simulink model "GPCA_AlarmNoActions"  (Simulink 9.0)
settings: Solver=FixedStepDiscrete  StartTime=0.0  StopTime=19.8  FixedStep=0.200000  RelTol=1e-3  EnableMultiTasking=on
model workspace (MAT data in the model file):
  already_pp = 1
  input_struct.time = [0; 0.2; 0.4; 0.6; 0.8; 1; 1.2; 1.4; 1.6; 1.8; 2; 2.2; 2.4; 2.6; 2.8; 3; 3.2; 3.4; 3.6; 3.8; 4; 4.2; 4.4; 4.6; 4.8; 5; 5.2; 5.4; 5.6; 5.8; 6; 6.2; 6.4; 6.6; 6.8; 7; 7.2; 7.4; 7.6; 7.8; 8; 8.2; 8.4; 8.6; 8.8; 9; 9.2; 9.4; 9.6; 9.8; 10; 10.2; 10.4; 10.6; 10.8; 11; 11.2; 11.4; 11.6; 11.8; 12; 12.2; 12.4; 12.6; 12.8; 13; 13.2; 13.4; 13.6; 13.8; 14; 14.2; 14.4; 14.6; 14.8; 15; 15.2; 15.4; 15.6; 15.8; 16; 16.2; 16.4; 16.6; 16.8; 17; 17.2; 17.4; 17.6; 17.8; 18; 18.2; 18.4; 18.6; 18.8; 19; 19.2; 19.4; 19.6; 19.8]
  input_struct.signals(1).name = 'In1'
  input_struct.signals(1).values = [1; 0; 1; 0; 0; 1; 0; 1; 0; 1; 1; 1; 0; 1; 1; 0; 0; 1; 1; 0; 0; 0; 0; 0; 0; 0; 0; 0; 1; 0; 1; 0; 0; 0; 1; 1; 1; 1; 1; 0; 0; 0; 0; 1; 1; 1; 1; 0; 1; 1; 0; 1; 1; 1; 1; 0; 0; 1; 0; 1; 1; 1; 0; 0; 0; 0; 1; 1; 1; 0; 0; 1; 0; 1; 1; 0; 1; 1; 1; 1; 1; 1; 1; 1; 0; 0; 1; 1; 0; 1; 1; 1; 0; 1; 1; 1; 1; 0; 1; 0]
  input_struct.signals(1).dimensions = 1
  input_struct.signals(2).name = 'In2'
  input_struct.signals(2).values = [0; 1; 1; 1; 0; 1; 0; 1; 1; 1; 0; 0; 0; 1; 1; 1; 1; 1; 0; 1; 0; 0; 1; 1; 1; 0; 1; 1; 0; 0; 0; 1; 0; 1; 1; 0; 0; 1; 1; 1; 1; 0; 0; 1; 1; 1; 0; 1; 0; 0; 0; 1; 0; 0; 0; 0; 1; 1; 0; 0; 1; 1; 1; 1; 0; 1; 0; 0; 0; 0; 0; 0; 0; 1; 0; 0; 1; 1; 1; 1; 1; 1; 1; 0; 0; 0; 0; 1; 0; 0; 1; 0; 1; 1; 1; 1; 0; 0; 1; 1]
  input_struct.signals(2).dimensions = 1
  input_struct.signals(3).name = 'In3'
  input_struct.signals(3).values = [1; 1; 1; 1; 0; 0; 0; 1; 1; 1; 1; 0; 1; 1; 0; 1; 1; 0; 1; 1; 0; 0; 0; 1; 1; 0; 1; 1; 1; 1; 0; 0; 1; 0; 0; 0; 1; 0; 1; 0; 1; 0; 0; 1; 0; 1; 1; 0; 0; 0; 0; 0; 1; 1; 1; 1; 0; 1; 0; 1; 0; 1; 0; 1; 1; 1; 1; 1; 0; 0; 1; 1; 1; 0; 1; 1; 0; 1; 1; 0; 1; 1; 0; 1; 1; 1; 1; 0; 0; 1; 1; 0; 0; 0; 0; 0; 1; 0; 0; 0]
  input_struct.signals(3).dimensions = 1
  input_struct.signals(4).name = 'In4'
  input_struct.signals(4).values = [0; 0; 0; 0; 0; 0; 0; 0; 0; 1; 0; 1; 0; 0; 0; 0; 0; 0; 0; 0; 0; 0; 1; 1; 1; 0; 0; 0; 1; 0; 0; 0; 0; 0; 1; 0; 1; 1; 0; 1; 1; 1; 1; 0; 1; 0; 0; 1; 1; 0; 0; 1; 1; 1; 1; 0; 1; 0; 1; 0; 1; 1; 0; 0; 0; 0; 0; 1; 0; 1; 0; 0; 0; 0; 1; 1; 1; 1; 0; 0; 0; 0; 0; 1; 1; 1; 0; 0; 1; 1; 1; 1; 1; 1; 0; 1; 0; 0; 0; 0]
  input_struct.signals(4).dimensions = 1
  input_struct.signals(5).name = 'In5'
  input_struct.signals(5).values = [1; 0; 1; 0; 0; 1; 0; 1; 1; 0; 0; 1; 1; 1; 0; 0; 1; 1; 1; 1; 1; 0; 1; 0; 0; 1; 0; 1; 1; 0; 0; 0; 1; 0; 0; 0; 0; 0; 0; 0; 0; 1; 0; 1; 1; 0; 0; 1; 0; 0; 1; 0; 1; 1; 1; 1; 0; 1; 0; 1; 1; 1; 0; 0; 0; 1; 1; 1; 1; 0; 1; 1; 0; 1; 0; 0; 1; 0; 1; 1; 1; 1; 1; 1; 0; 0; 1; 0; 0; 0; 1; 1; 1; 0; 0; 1; 1; 1; 0; 0]
  input_struct.signals(5).dimensions = 1
  input_struct.signals(6).name = 'In6'
  input_struct.signals(6).values = [1; 1; 1; 0; 1; 0; 1; 0; 0; 0; 1; 1; 0; 0; 0; 1; 1; 0; 0; 0; 1; 1; 0; 0; 1; 0; 0; 1; 0; 1; 1; 1; 0; 1; 1; 0; 1; 0; 0; 0; 1; 1; 0; 1; 0; 1; 1; 0; 1; 0; 1; 0; 0; 1; 1; 0; 0; 1; 0; 1; 1; 1; 0; 0; 1; 1; 1; 1; 1; 0; 1; 0; 0; 0; 1; 1; 1; 1; 1; 1; 1; 0; 0; 0; 1; 1; 1; 1; 0; 1; 1; 0; 1; 0; 0; 0; 0; 1; 0; 0]
  input_struct.signals(6).dimensions = 1
  input_struct.signals(7).name = 'In7'
  input_struct.signals(7).values = [0; 0; 0; 1; 0; 0; 0; 1; 0; 1; 1; 0; 1; 1; 0; 1; 1; 0; 0; 1; 1; 1; 0; 1; 1; 1; 1; 0; 0; 0; 0; 0; 0; 1; 1; 0; 0; 0; 0; 0; 0; 1; 0; 1; 0; 0; 0; 0; 0; 1; 0; 1; 1; 1; 0; 0; 0; 1; 1; 0; 0; 1; 1; 0; 1; 1; 0; 1; 0; 0; 1; 1; 0; 1; 1; 1; 0; 0; 0; 1; 0; 0; 1; 1; 0; 0; 0; 1; 0; 0; 1; 0; 1; 1; 0; 0; 1; 1; 1; 1]
  input_struct.signals(7).dimensions = 1
  input_struct.signals(8).name = 'In8'
  input_struct.signals(8).values = [0; 1; 0; 0; 0; 1; 1; 1; 1; 0; 1; 0; 1; 1; 1; 0; 0; 1; 1; 1; 1; 1; 1; 1; 0; 1; 0; 0; 1; 0; 0; 1; 0; 0; 0; 0; 0; 1; 0; 0; 0; 0; 1; 0; 1; 1; 1; 1; 0; 0; 1; 0; 1; 1; 1; 0; 1; 0; 0; 0; 1; 1; 1; 1; 0; 1; 0; 1; 1; 1; 1; 1; 0; 0; 1; 0; 0; 0; 0; 1; 1; 1; 0; 1; 1; 1; 1; 0; 1; 0; 1; 1; 1; 0; 1; 0; 0; 1; 1; 0]
  input_struct.signals(8).dimensions = 1
  input_struct.signals(9).name = 'In9'
  input_struct.signals(9).values = [1; 1; 0; 0; 0; 0; 0; 1; 0; 1; 0; 1; 0; 1; 1; 0; 0; 0; 0; 0; 0; 1; 1; 1; 0; 1; 0; 1; 1; 0; 1; 1; 1; 1; 1; 0; 0; 0; 1; 1; 0; 0; 1; 1; 1; 0; 1; 1; 0; 0; 0; 1; 1; 0; 1; 1; 0; 0; 1; 1; 1; 1; 0; 0; 1; 1; 1; 0; 1; 1; 1; 0; 0; 1; 0; 1; 1; 0; 1; 0; 1; 0; 0; 1; 0; 0; 0; 0; 1; 1; 0; 0; 1; 0; 1; 1; 1; 1; 0; 1]
  input_struct.signals(9).dimensions : numeric (value not decoded)
settings Model: SuppressorTable=22 serialization::archive 11 0 6 0 0 0 0 0  Creator=bourbouh  LastModifiedBy=hbourbou
settings DataIOCC: ExternalInput=input_struct  LoadExternalInput=on  SaveFormat=Structure  SaveState=on
settings DebuggingCC: AlgebraicLoopMsg=error  ArtificialAlgebraicLoopMsg=error  UnderspecifiedInitializationDetection=Simplified  MergeDetectMultiDrivingBlocksExec=error  SingleTaskRateTransMsg=error
settings HardwareCC: ProdBitPerPointer=64  ProdBitPerSizeT=64  ProdBitPerPtrDiffT=64  ProdLargestAtomicFloat=Float  ProdIntDivRoundTo=Zero  ProdEndianess=LittleEndian  ProdWordSize=64  ProdHWDeviceType=Intel->x86-64 (Windows64)
settings ModelReferenceCC: PropagateSignalLabelsOutOfModel=on
settings GRTTargetCC: GeneratePreprocessorConditionals=Disable all  ExtMode=on

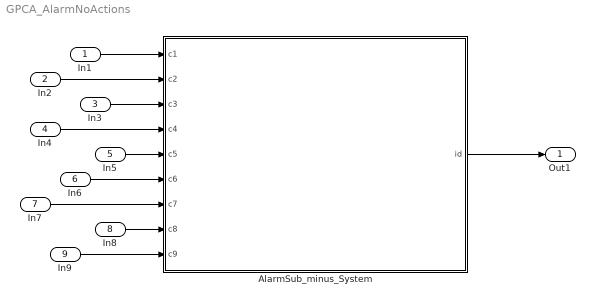
== system GPCA_AlarmNoActions ==
  In1 : Inport  OutDataTypeStr=boolean  PortDimensions=1
  In2 : Inport  Port=2  OutDataTypeStr=boolean  PortDimensions=1
  In3 : Inport  Port=3  OutDataTypeStr=boolean  PortDimensions=1
  In4 : Inport  Port=4  OutDataTypeStr=boolean  PortDimensions=1
  In5 : Inport  Port=5  OutDataTypeStr=boolean  PortDimensions=1
  In6 : Inport  Port=6  OutDataTypeStr=boolean  PortDimensions=1
  In7 : Inport  Port=7  OutDataTypeStr=boolean  PortDimensions=1
  In8 : Inport  Port=8  OutDataTypeStr=boolean  PortDimensions=1
  In9 : Inport  Port=9  OutDataTypeStr=boolean  PortDimensions=1
  AlarmSub_minus_System : Stateflow chart  TreatAsAtomicUnit=on
  Out1 : Outport
  wires:
  AlarmSub_minus_System/1(id) -> Out1/1
  In9/1 -> AlarmSub_minus_System/9(c9)
  In8/1 -> AlarmSub_minus_System/8(c8)
  In7/1 -> AlarmSub_minus_System/7(c7)
  In6/1 -> AlarmSub_minus_System/6(c6)
  In5/1 -> AlarmSub_minus_System/5(c5)
  In4/1 -> AlarmSub_minus_System/4(c4)
  In3/1 -> AlarmSub_minus_System/3(c3)
  In2/1 -> AlarmSub_minus_System/2(c2)
  In1/1 -> AlarmSub_minus_System/1(c1)

== stateflow chart AlarmSub_minus_System ==
  state Alarms
    state CheckAlarm [parallel]
      settings: executionOrder=1
      state CancelAlarm [parallel]
        settings: executionOrder=1
        state ON
          en: id = 2112;
        state OFF
          en: id = 2111;
        (default) -> Alarms.CheckAlarm.CancelAlarm.OFF
        Alarms.CheckAlarm.CancelAlarm.OFF -> Alarms.CheckAlarm.CancelAlarm.ON : [c5]
        Alarms.CheckAlarm.CancelAlarm.ON -> Alarms.CheckAlarm.CancelAlarm.OFF : [c4]
      state Level4 [parallel]
        settings: executionOrder=2
        state IsEmptyReservoir [parallel]
          settings: executionOrder=1
          state No
            en: id=21111;
          state Yes
            en: id=21112;
          (default) -> Alarms.CheckAlarm.Level4.IsEmptyReservoir.No [order 2]
          (default) -> Alarms.CheckAlarm.Level4.IsEmptyReservoir.Yes [order 1] : [c6]
          Alarms.CheckAlarm.Level4.IsEmptyReservoir.No -> Alarms.CheckAlarm.Level4.IsEmptyReservoir.Yes : [c7]
          Alarms.CheckAlarm.Level4.IsEmptyReservoir.Yes -> Alarms.CheckAlarm.Level4.IsEmptyReservoir.No [order 2] : [c8]
          Alarms.CheckAlarm.Level4.IsEmptyReservoir.Yes -> Alarms.CheckAlarm.Level4.IsEmptyReservoir.Yes [order 1] : [c9]
        state IsHardwareError [parallel]
          settings: executionOrder=2
          state Yes
            en: id=21122;
          state No
            en: id=21121;
          (default) -> Alarms.CheckAlarm.Level4.IsHardwareError.No [order 2]
          (default) -> Alarms.CheckAlarm.Level4.IsHardwareError.Yes [order 1] : [c3]
          Alarms.CheckAlarm.Level4.IsHardwareError.No -> Alarms.CheckAlarm.Level4.IsHardwareError.Yes : [c2]
          Alarms.CheckAlarm.Level4.IsHardwareError.Yes -> Alarms.CheckAlarm.Level4.IsHardwareError.No : [c4]
        state IsEnviromentalError [parallel]
          settings: executionOrder=3
          state Yes
            en: id=21132;
          state No
            en: id=21131;
          (default) -> Alarms.CheckAlarm.Level4.IsEnviromentalError.Yes [order 1] : [c6]
          (default) -> Alarms.CheckAlarm.Level4.IsEnviromentalError.No [order 2]
          Alarms.CheckAlarm.Level4.IsEnviromentalError.No -> Alarms.CheckAlarm.Level4.IsEnviromentalError.Yes : [c5]
          Alarms.CheckAlarm.Level4.IsEnviromentalError.Yes -> Alarms.CheckAlarm.Level4.IsEnviromentalError.No : [c7]
      state Level3 [parallel]
        settings: executionOrder=3
        state IsOverInfusionFlowRate [parallel]
          entry:id=21131;
          settings: executionOrder=1
          state Yes
            entry:id=21133;
          state Check
            entry:id=21132;
          state Monitor
            entry:id=21134;
          (default) -> Alarms.CheckAlarm.Level3.IsOverInfusionFlowRate.Check [order 3]
          (default) -> Alarms.CheckAlarm.Level3.IsOverInfusionFlowRate.Yes [order 1] : [c4]
          Alarms.CheckAlarm.Level3.IsOverInfusionFlowRate.Yes -> Alarms.CheckAlarm.Level3.IsOverInfusionFlowRate.Yes [order 1] : [c5]
          Alarms.CheckAlarm.Level3.IsOverInfusionFlowRate.Check -> Alarms.CheckAlarm.Level3.IsOverInfusionFlowRate.Yes [order 1] : [c6]
          Alarms.CheckAlarm.Level3.IsOverInfusionFlowRate.Yes -> Alarms.CheckAlarm.Level3.IsOverInfusionFlowRate.Check [order 2] : [c7]
          Alarms.CheckAlarm.Level3.IsOverInfusionFlowRate.Monitor -> Alarms.CheckAlarm.Level3.IsOverInfusionFlowRate.Yes [order 1] : [c7]
          Alarms.CheckAlarm.Level3.IsOverInfusionFlowRate.Monitor -> Alarms.CheckAlarm.Level3.IsOverInfusionFlowRate.Check [order 2] : [c9]
          Alarms.CheckAlarm.Level3.IsOverInfusionFlowRate.Check -> Alarms.CheckAlarm.Level3.IsOverInfusionFlowRate.Monitor [order 2] : [c8]
          Alarms.CheckAlarm.Level3.IsOverInfusionFlowRate.Monitor -> Alarms.CheckAlarm.Level3.IsOverInfusionFlowRate.Monitor [order 3] : [c8]
          (default) -> Alarms.CheckAlarm.Level3.IsOverInfusionFlowRate.Monitor [order 2] : [c4]
        state IsOverInfusionVTBI [parallel]
          settings: executionOrder=2
          state Yes
            en: id=211342
          state No
            en: id = 211341;
          (default) -> Alarms.CheckAlarm.Level3.IsOverInfusionVTBI.No [order 2]
          (default) -> Alarms.CheckAlarm.Level3.IsOverInfusionVTBI.Yes [order 1] : [c5]
          Alarms.CheckAlarm.Level3.IsOverInfusionVTBI.Yes -> Alarms.CheckAlarm.Level3.IsOverInfusionVTBI.Yes [order 1] : [c6]
          Alarms.CheckAlarm.Level3.IsOverInfusionVTBI.No -> Alarms.CheckAlarm.Level3.IsOverInfusionVTBI.Yes : [c7]
          Alarms.CheckAlarm.Level3.IsOverInfusionVTBI.Yes -> Alarms.CheckAlarm.Level3.IsOverInfusionVTBI.No [order 2] : [c8]
        state IsAirInLine [parallel]
          settings: executionOrder=3
          state Yes
            en: id=211332
          state No
            en: id = 211331;
          (default) -> Alarms.CheckAlarm.Level3.IsAirInLine.Yes [order 1] : [c1]
          (default) -> Alarms.CheckAlarm.Level3.IsAirInLine.No [order 2]
          Alarms.CheckAlarm.Level3.IsAirInLine.No -> Alarms.CheckAlarm.Level3.IsAirInLine.Yes : [c2]
          Alarms.CheckAlarm.Level3.IsAirInLine.Yes -> Alarms.CheckAlarm.Level3.IsAirInLine.No : [c3]
        state IsOcclusion [parallel]
          settings: executionOrder=4
          state Yes
            en: id=31132
          state No
            en: id=31131
          (default) -> Alarms.CheckAlarm.Level3.IsOcclusion.No [order 2]
          (default) -> Alarms.CheckAlarm.Level3.IsOcclusion.Yes [order 1] : [c7]
          Alarms.CheckAlarm.Level3.IsOcclusion.No -> Alarms.CheckAlarm.Level3.IsOcclusion.Yes : [c8]
          Alarms.CheckAlarm.Level3.IsOcclusion.Yes -> Alarms.CheckAlarm.Level3.IsOcclusion.No : [c9]
        state IsDoor_Open [parallel]
          settings: executionOrder=5
          state No
            en: id=32221
          state Yes
            en: id=32222
          (default) -> Alarms.CheckAlarm.Level3.IsDoor_Open.Yes [order 1] : [c1]
          (default) -> Alarms.CheckAlarm.Level3.IsDoor_Open.No [order 2]
          Alarms.CheckAlarm.Level3.IsDoor_Open.No -> Alarms.CheckAlarm.Level3.IsDoor_Open.Yes : [c2]
          Alarms.CheckAlarm.Level3.IsDoor_Open.Yes -> Alarms.CheckAlarm.Level3.IsDoor_Open.No : [c3]
      state Level2 [parallel]
        settings: executionOrder=4
        state IsLowReservoir [parallel]
          settings: executionOrder=1
          state No
            en: id = 42421;
          state Yes
            en: id=42422;
          (default) -> Alarms.CheckAlarm.Level2.IsLowReservoir.Yes [order 1] : [c5]
          (default) -> Alarms.CheckAlarm.Level2.IsLowReservoir.No [order 2]
          Alarms.CheckAlarm.Level2.IsLowReservoir.No -> Alarms.CheckAlarm.Level2.IsLowReservoir.Yes : [c6]
          Alarms.CheckAlarm.Level2.IsLowReservoir.Yes -> Alarms.CheckAlarm.Level2.IsLowReservoir.No : [c7]
      state Level1 [parallel]
        settings: executionOrder=5
        state IsUnderInfusion [parallel]
          entry: id=55111;
          settings: executionOrder=1
          state Yes
            entry:id=55113;
          state Check
            entry: id=55112;
          state Monitor
            entry: id=55114;
          (default) -> Alarms.CheckAlarm.Level1.IsUnderInfusion.Check [order 3]
          (default) -> Alarms.CheckAlarm.Level1.IsUnderInfusion.Yes [order 1] : [c1]
          Alarms.CheckAlarm.Level1.IsUnderInfusion.Check -> Alarms.CheckAlarm.Level1.IsUnderInfusion.Yes [order 1] : [c8]
          Alarms.CheckAlarm.Level1.IsUnderInfusion.Yes -> Alarms.CheckAlarm.Level1.IsUnderInfusion.Check : [c9]
          Alarms.CheckAlarm.Level1.IsUnderInfusion.Monitor -> Alarms.CheckAlarm.Level1.IsUnderInfusion.Yes [order 1] : [c2]
          Alarms.CheckAlarm.Level1.IsUnderInfusion.Monitor -> Alarms.CheckAlarm.Level1.IsUnderInfusion.Check [order 3] : [c6]
          Alarms.CheckAlarm.Level1.IsUnderInfusion.Check -> Alarms.CheckAlarm.Level1.IsUnderInfusion.Monitor [order 2] : [c5]
          (default) -> Alarms.CheckAlarm.Level1.IsUnderInfusion.Monitor [order 2] : [c3]
          Alarms.CheckAlarm.Level1.IsUnderInfusion.Monitor -> Alarms.CheckAlarm.Level1.IsUnderInfusion.Monitor [order 2] : [c4]
        state IsFlowRateNotStable [parallel]
          settings: executionOrder=2
          state Yes
            en: id=55122;
          state No
            en: id=55121;
          (default) -> Alarms.CheckAlarm.Level1.IsFlowRateNotStable.Yes [order 1] : [c8]
          (default) -> Alarms.CheckAlarm.Level1.IsFlowRateNotStable.No [order 2]
          Alarms.CheckAlarm.Level1.IsFlowRateNotStable.No -> Alarms.CheckAlarm.Level1.IsFlowRateNotStable.Yes : [c5]
          Alarms.CheckAlarm.Level1.IsFlowRateNotStable.Yes -> Alarms.CheckAlarm.Level1.IsFlowRateNotStable.No : [c6]
        state IsPausedTimeExceeded [parallel]
          settings: executionOrder=4
          state counting
            entry: id=43342;
          state No
            entry:id=43341;
          state Yes
            en: id=43343;
          (default) -> Alarms.CheckAlarm.Level1.IsPausedTimeExceeded.counting [order 2] : [c8 ]{}
          (default) -> Alarms.CheckAlarm.Level1.IsPausedTimeExceeded.No [order 3]
          Alarms.CheckAlarm.Level1.IsPausedTimeExceeded.No -> Alarms.CheckAlarm.Level1.IsPausedTimeExceeded.counting [order 2] : [c7]
          Alarms.CheckAlarm.Level1.IsPausedTimeExceeded.Yes -> Alarms.CheckAlarm.Level1.IsPausedTimeExceeded.No : [c1]
          Alarms.CheckAlarm.Level1.IsPausedTimeExceeded.No -> Alarms.CheckAlarm.Level1.IsPausedTimeExceeded.Yes [order 1] : [c2]
          Alarms.CheckAlarm.Level1.IsPausedTimeExceeded.counting -> Alarms.CheckAlarm.Level1.IsPausedTimeExceeded.Yes : [ c9]
          (default) -> Alarms.CheckAlarm.Level1.IsPausedTimeExceeded.Yes [order 1] : [c3]
        state IsIdleTimeExceeded [parallel]
          settings: executionOrder=3
          state counting
            entry: id=56232;
          state No
            entry:id=56231;
          state Yes
            en: id=56233;
          (default) -> Alarms.CheckAlarm.Level1.IsIdleTimeExceeded.counting [order 2] : [c5]{}
          (default) -> Alarms.CheckAlarm.Level1.IsIdleTimeExceeded.No [order 3]
          Alarms.CheckAlarm.Level1.IsIdleTimeExceeded.No -> Alarms.CheckAlarm.Level1.IsIdleTimeExceeded.counting [order 2] : [c4]
          Alarms.CheckAlarm.Level1.IsIdleTimeExceeded.Yes -> Alarms.CheckAlarm.Level1.IsIdleTimeExceeded.No : [c1]
          Alarms.CheckAlarm.Level1.IsIdleTimeExceeded.No -> Alarms.CheckAlarm.Level1.IsIdleTimeExceeded.Yes [order 1] : [c2]
          Alarms.CheckAlarm.Level1.IsIdleTimeExceeded.counting -> Alarms.CheckAlarm.Level1.IsIdleTimeExceeded.Yes : [c3]
          (default) -> Alarms.CheckAlarm.Level1.IsIdleTimeExceeded.Yes [order 1] : [c7]
        state IsConfigTimeWarning [parallel]
          settings: executionOrder=5
          state No
            en: id=53241;
          state Yes
            en: id=43242;
          (default) -> Alarms.CheckAlarm.Level1.IsConfigTimeWarning.No [order 2]
          (default) -> Alarms.CheckAlarm.Level1.IsConfigTimeWarning.Yes [order 1] : [c7]
          Alarms.CheckAlarm.Level1.IsConfigTimeWarning.No -> Alarms.CheckAlarm.Level1.IsConfigTimeWarning.Yes : [c8]
          Alarms.CheckAlarm.Level1.IsConfigTimeWarning.Yes -> Alarms.CheckAlarm.Level1.IsConfigTimeWarning.No : [c9]
        state IsBatteryError [parallel]
          settings: executionOrder=6
          state Yes
            en: id=72772;
          state No
            en: id=72771;
          (default) -> Alarms.CheckAlarm.Level1.IsBatteryError.Yes [order 1] : [c5]
          (default) -> Alarms.CheckAlarm.Level1.IsBatteryError.No [order 2]
          Alarms.CheckAlarm.Level1.IsBatteryError.No -> Alarms.CheckAlarm.Level1.IsBatteryError.Yes : [c6]
          Alarms.CheckAlarm.Level1.IsBatteryError.Yes -> Alarms.CheckAlarm.Level1.IsBatteryError.No : [c7]
        state IsPumpHot [parallel]
          settings: executionOrder=7
          state Yes
            en: id=92372;
          state No
            en: id=92371;
          (default) -> Alarms.CheckAlarm.Level1.IsPumpHot.Yes [order 1] : [c1]
          (default) -> Alarms.CheckAlarm.Level1.IsPumpHot.No [order 2]
          Alarms.CheckAlarm.Level1.IsPumpHot.No -> Alarms.CheckAlarm.Level1.IsPumpHot.Yes : [c4]
          Alarms.CheckAlarm.Level1.IsPumpHot.Yes -> Alarms.CheckAlarm.Level1.IsPumpHot.No : [ c2]
        state IsLoggingFailed [parallel]
          settings: executionOrder=8
          state Yes
            en: id=32382;
          state No
            en: id=32381;
          (default) -> Alarms.CheckAlarm.Level1.IsLoggingFailed.Yes [order 1] : [c4 ]
          (default) -> Alarms.CheckAlarm.Level1.IsLoggingFailed.No [order 2]
          Alarms.CheckAlarm.Level1.IsLoggingFailed.No -> Alarms.CheckAlarm.Level1.IsLoggingFailed.Yes : [c5 ]
          Alarms.CheckAlarm.Level1.IsLoggingFailed.Yes -> Alarms.CheckAlarm.Level1.IsLoggingFailed.No : [c6]
        state IsSystemMonitorFailed [parallel]
          settings: executionOrder=9
          state Yes
            en: id=42492;
          state No
            en: id=42491;
          (default) -> Alarms.CheckAlarm.Level1.IsSystemMonitorFailed.Yes [order 1] : [c1]
          (default) -> Alarms.CheckAlarm.Level1.IsSystemMonitorFailed.No [order 2]
          Alarms.CheckAlarm.Level1.IsSystemMonitorFailed.No -> Alarms.CheckAlarm.Level1.IsSystemMonitorFailed.Yes : [c2]
          Alarms.CheckAlarm.Level1.IsSystemMonitorFailed.Yes -> Alarms.CheckAlarm.Level1.IsSystemMonitorFailed.No : [c3]
      state SetAlarmStatus [parallel]
        entry: id = 216;
        settings: executionOrder=6
    state Notification [parallel]
      settings: executionOrder=2
      state Visual [parallel]
        settings: executionOrder=1
        state OFF
          entry:id=2211;
        state AlarmDisplay
          entry:id=2212;
        (default) -> Alarms.Notification.Visual.OFF [order 2]
        (default) -> AlarmDisplay [order 1] : [c2]
        Alarms.Notification.Visual.OFF -> AlarmDisplay : [c3]
        AlarmDisplay -> Alarms.Notification.Visual.OFF [order 1] : [c4]
        AlarmDisplay -> AlarmDisplay [order 2] : [c1]
      state Audio [parallel]
        entry: id=22220;
        settings: executionOrder=2
        state Disabled
          entry: id=2224;
        state Silenced
          entry: id=2223;
        state OFF
          entry: id=2221;
        state ON
          entry: id=2222;
        (default) -> Alarms.Notification.Audio.OFF [order 4]
        Alarms.Notification.Audio.ON -> Alarms.Notification.Audio.ON [order 3] : [c7]
        (default) -> Alarms.Notification.Audio.ON [order 3] : [c6]
        Alarms.Notification.Audio.OFF -> Alarms.Notification.Audio.ON [order 3] : [c1]
        Alarms.Notification.Audio.ON -> Alarms.Notification.Audio.OFF [order 4] : [c4]
        (junction 182) -> Alarms.Notification.Audio.ON : [c5]
        Alarms.Notification.Audio.OFF -> Disabled [order 1] : [c3]
        (junction 181) -> Alarms.Notification.Audio.OFF
        Alarms.Notification.Audio.OFF -> (junction 180) [order 2]
        Alarms.Notification.Audio.ON -> (junction 180) [order 2]
        Alarms.Notification.Audio.ON -> Disabled [order 1] : [c1]
        (junction 180) -> Silenced : [c7]
        Silenced -> (junction 181) [order 3] : [c7]
        Silenced -> (junction 182) [order 2] : [c9]
        Disabled -> (junction 181) [order 3] : [c1]
        Disabled -> (junction 182) [order 2] : [c5]
        Silenced -> Disabled [order 1] : [c8]
        (default) -> Silenced [order 2] : [c3]
        Disabled -> Silenced [order 1] : [c2]
        (default) -> Disabled [order 1] : [c4]
  state NOT_ON
    en: id = 1;
  (default) -> Alarms [order 1] : [c1]
  (default) -> NOT_ON [order 2]
  NOT_ON -> Alarms : [c7]
  Alarms -> NOT_ON : [c8]
  data: id output double; c1 input boolean; c2 input boolean; c3 input boolean; c4 input boolean; c5 input boolean; c6 input boolean; c7 input boolean; c8 input boolean; c9 input boolean
